simulink model "dcm_to_q"  (R2021b)
settings: Solver=VariableStepAuto  StartTime=0.0  StopTime=10.0  RelTol=1e-3
undefined symbols (not defined in the file): A_dcm
settings Model: Creator=jorgemarrero  LastModifiedBy=jorgemarrero

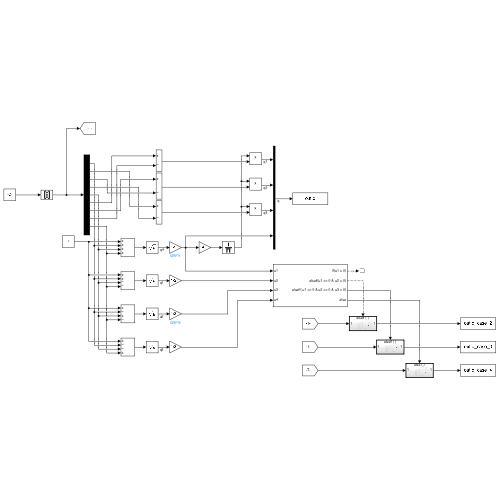
[thumbnail: Simulink's stored preview of the top-level diagram]
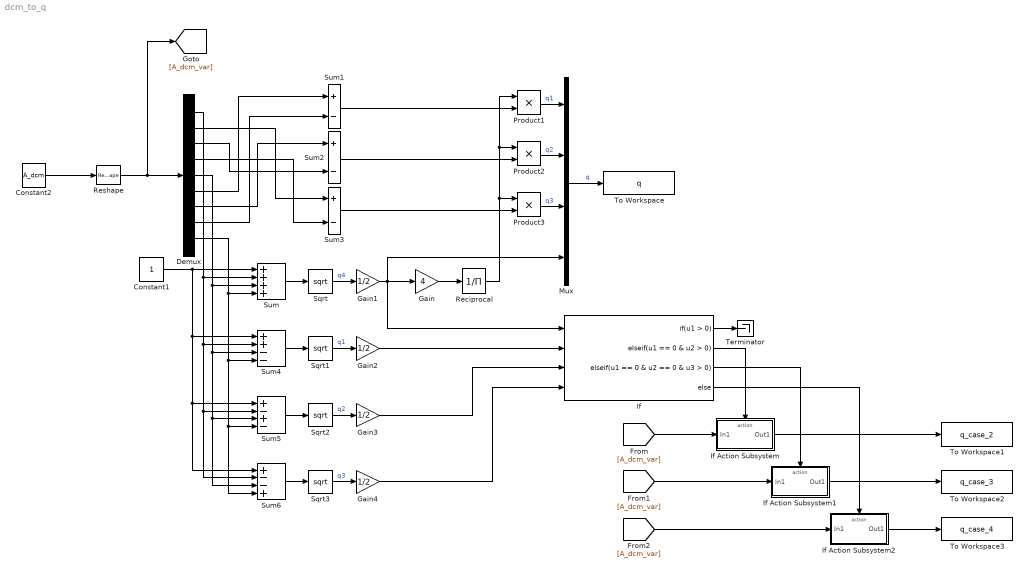
== system dcm_to_q ==
  Constant1 : Constant
  Constant2 : Constant  Value=A_dcm
  Demux : Demux  Outputs=9
  Gain : Gain  Gain=4
  Gain{1..4} (4 alike) : Gain  Gain=1/2
  If : If  NumInputs=4  ElseIfExpressions=u1 == 0 & u2 > 0, u1 == 0 & u2 == 0 & u3 > 0
  If Action Subsystem : Subsystem  TreatAsAtomicUnit=on
  If Action Subsystem1 : Subsystem  TreatAsAtomicUnit=on
  If Action Subsystem2 : Subsystem  TreatAsAtomicUnit=on
  Mux : Mux
  Product1 : Product
  Product2 : Product
  Product3 : Product
  Reciprocal : Product  Inputs=/
  Reshape : Reshape  OutputDimensionality=Column vector (2-D)
  Sqrt{,1..3} (4 alike) : Sqrt  SaturateOnIntegerOverflow=on
  Sum : Sum  Inputs=++++
  Sum1 : Sum  Inputs=+-
  Sum2 : Sum  Inputs=+-
  Sum3 : Sum  Inputs=+-
  Sum4 : Sum  Inputs=++--
  Sum5 : Sum  Inputs=+-+-
  Sum6 : Sum  Inputs=+--+
  Terminator : Terminator
  To Workspace : ToWorkspace  VariableName=q  SaveFormat=Timeseries  SampleTime=-1
  To Workspace1 : ToWorkspace  VariableName=q_case_2  SaveFormat=Timeseries  SampleTime=-1
  To Workspace2 : ToWorkspace  VariableName=q_case_3  SaveFormat=Timeseries  SampleTime=-1
  To Workspace3 : ToWorkspace  VariableName=q_case_4  SaveFormat=Timeseries  SampleTime=-1
  wires:
  Constant2/1 -> Reshape/1
  Sum/1 -> Sqrt/1
  Sum1/1 -> Product1/2
  Product1/1 -> Mux/1  "q1"
  Product2/1 -> Mux/2  "q2"
  Sum2/1 -> Product2/2
  Sum3/1 -> Product3/2
  Product3/1 -> Mux/3  "q3"
  Mux/1 -> To Workspace/1  "q"
  If/1 -> Terminator/1
  If/2 -> If Action Subsystem/Action
  Sum4/1 -> Sqrt1/1
  Demux/5 -> Sum6/3, Sum5/3, Sum4/3, Sum/3
  Constant1/1 -> Sum6/1, Sum5/1, Sum4/1, Sum/1
  Demux/9 -> Sum6/4, Sum5/4, Sum4/4, Sum/4
  Demux/1 -> Sum6/2, Sum5/2, Sum4/2, Sum/2
  Reshape/1 -> [A_dcm_var], Demux/1
  [A_dcm_var] -> If Action Subsystem/1(In1)
  Sqrt/1 -> Gain1/1  "q4"
  Gain/1 -> Reciprocal/1
  Reciprocal/1 -> Product3/1, Product2/1, Product1/1
  Sum5/1 -> Sqrt2/1
  Sum6/1 -> Sqrt3/1
  Gain1/1 -> If/1, Gain/1, Mux/4
  Sqrt1/1 -> Gain2/1  "q1"
  Sqrt2/1 -> Gain3/1  "q2"
  Sqrt3/1 -> Gain4/1  "q3"
  Gain2/1 -> If/2
  Gain3/1 -> If/3
  Gain4/1 -> If/4
  [A_dcm_var] -> If Action Subsystem1/1(In1)
  [A_dcm_var] -> If Action Subsystem2/1(In1)
  Demux/6 -> Sum1/1
  Demux/8 -> Sum1/2
  Demux/7 -> Sum2/1
  Demux/3 -> Sum2/2
  Demux/2 -> Sum3/1
  Demux/4 -> Sum3/2
  If Action Subsystem/1(Out1) -> To Workspace1/1
  If Action Subsystem1/1(Out1) -> To Workspace2/1
  If Action Subsystem2/1(Out1) -> To Workspace3/1
  If/3 -> If Action Subsystem1/Action
  If/4 -> If Action Subsystem2/Action

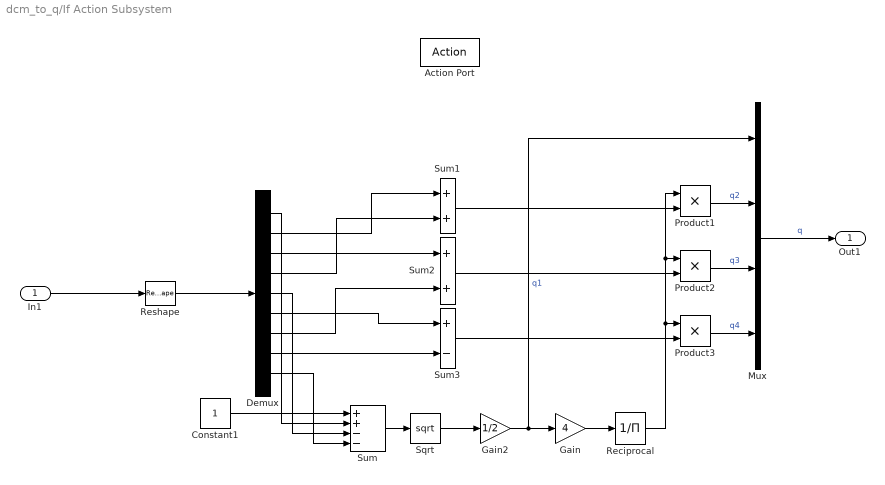
== system dcm_to_q/If Action Subsystem ==
  In1 : Inport
  Action Port : ActionPort  ActionPortLabel=elseif(u1 == 0 & u2 > 0)
  Constant1 : Constant
  Demux : Demux  Outputs=9
  Gain : Gain  Gain=4
  Gain2 : Gain  Gain=1/2
  Mux : Mux
  Product1 : Product
  Product2 : Product
  Product3 : Product
  Reciprocal : Product  Inputs=/
  Reshape : Reshape  OutputDimensionality=Column vector (2-D)
  Sqrt : Sqrt  SaturateOnIntegerOverflow=on
  Sum : Sum  Inputs=++--
  Sum1 : Sum
  Sum2 : Sum
  Sum3 : Sum  Inputs=+-
  Out1 : Outport
  wires:
  Sum2/1 -> Product2/2
  Demux/5 -> Sum/3
  Sum1/1 -> Product1/2
  Demux/3 -> Sum2/1
  Demux/8 -> Sum3/2
  Demux/6 -> Sum3/1
  Demux/2 -> Sum1/1
  Demux/4 -> Sum1/2
  Sum/1 -> Sqrt/1
  Demux/9 -> Sum/4
  Demux/7 -> Sum2/2
  Sum3/1 -> Product3/2
  Constant1/1 -> Sum/1
  Demux/1 -> Sum/2
  In1/1 -> Reshape/1
  Mux/1 -> Out1/1  "q"
  Reshape/1 -> Demux/1
  Reciprocal/1 -> Product1/1, Product2/1, Product3/1
  Product1/1 -> Mux/2  "q2"
  Product3/1 -> Mux/4  "q4"
  Product2/1 -> Mux/3  "q3"
  Gain2/1 -> Mux/1, Gain/1  "q1"
  Sqrt/1 -> Gain2/1
  Gain/1 -> Reciprocal/1

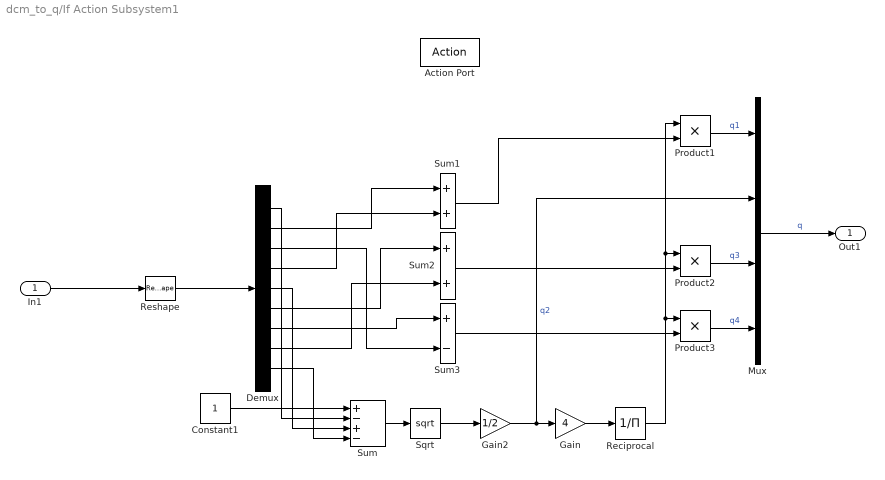
== system dcm_to_q/If Action Subsystem1 ==
  In1 : Inport
  Action Port : ActionPort  ActionPortLabel=elseif( u1 == 0 & u2 == 0 & u3 > 0)
  Constant1 : Constant
  Demux : Demux  Outputs=9
  Gain : Gain  Gain=4
  Gain2 : Gain  Gain=1/2
  Mux : Mux
  Product1 : Product
  Product2 : Product
  Product3 : Product
  Reciprocal : Product  Inputs=/
  Reshape : Reshape  OutputDimensionality=Column vector (2-D)
  Sqrt : Sqrt  SaturateOnIntegerOverflow=on
  Sum : Sum  Inputs=+-+-
  Sum1 : Sum
  Sum2 : Sum
  Sum3 : Sum  Inputs=+-
  Out1 : Outport
  wires:
  Demux/9 -> Sum/4
  Reciprocal/1 -> Product1/1, Product2/1, Product3/1
  Demux/5 -> Sum/3
  Reshape/1 -> Demux/1
  Sum1/1 -> Product1/2
  Constant1/1 -> Sum/1
  Sum2/1 -> Product2/2
  Sum3/1 -> Product3/2
  In1/1 -> Reshape/1
  Demux/4 -> Sum1/2
  Demux/2 -> Sum1/1
  Sqrt/1 -> Gain2/1
  Gain/1 -> Reciprocal/1
  Mux/1 -> Out1/1  "q"
  Demux/1 -> Sum/2
  Product2/1 -> Mux/3  "q3"
  Product3/1 -> Mux/4  "q4"
  Gain2/1 -> Mux/2, Gain/1  "q2"
  Sum/1 -> Sqrt/1
  Product1/1 -> Mux/1  "q1"
  Demux/6 -> Sum2/1
  Demux/8 -> Sum2/2
  Demux/7 -> Sum3/1
  Demux/3 -> Sum3/2

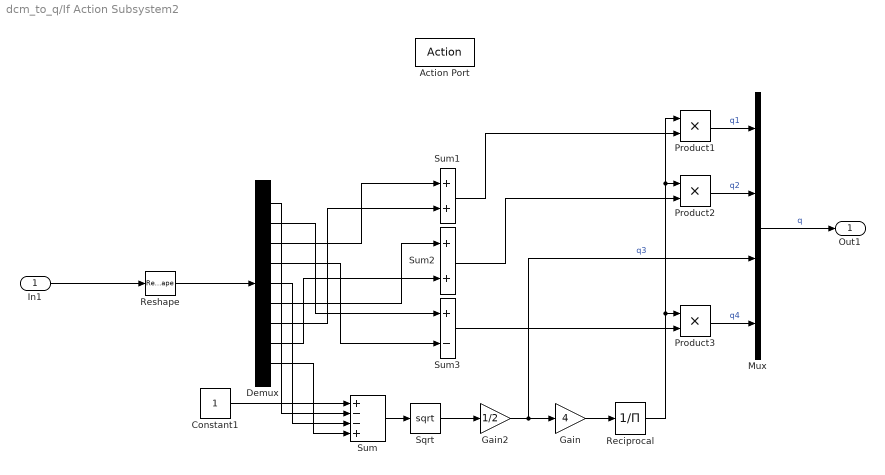
== system dcm_to_q/If Action Subsystem2 ==
  In1 : Inport
  Action Port : ActionPort  ActionPortLabel=else
  Constant1 : Constant
  Demux : Demux  Outputs=9
  Gain : Gain  Gain=4
  Gain2 : Gain  Gain=1/2
  Mux : Mux
  Product1 : Product
  Product2 : Product
  Product3 : Product
  Reciprocal : Product  Inputs=/
  Reshape : Reshape  OutputDimensionality=Column vector (2-D)
  Sqrt : Sqrt  SaturateOnIntegerOverflow=on
  Sum : Sum  Inputs=+--+
  Sum1 : Sum
  Sum2 : Sum
  Sum3 : Sum  Inputs=+-
  Out1 : Outport
  wires:
  Reciprocal/1 -> Product1/1, Product2/1, Product3/1
  Product3/1 -> Mux/4  "q4"
  Demux/1 -> Sum/2
  Product1/1 -> Mux/1  "q1"
  Sqrt/1 -> Gain2/1
  Gain/1 -> Reciprocal/1
  Mux/1 -> Out1/1  "q"
  Constant1/1 -> Sum/1
  In1/1 -> Reshape/1
  Sum2/1 -> Product2/2
  Reshape/1 -> Demux/1
  Sum3/1 -> Product3/2
  Sum1/1 -> Product1/2
  Demux/5 -> Sum/3
  Demux/9 -> Sum/4
  Gain2/1 -> Mux/3, Gain/1  "q3"
  Sum/1 -> Sqrt/1
  Product2/1 -> Mux/2  "q2"
  Demux/3 -> Sum1/1
  Demux/7 -> Sum1/2
  Demux/6 -> Sum2/1
  Demux/8 -> Sum2/2
  Demux/2 -> Sum3/1
  Demux/4 -> Sum3/2
